simulink model "dspanc"  (Simulink 6.0)
settings: Solver=FixedStepDiscrete  StartTime=0.0  StopTime=7.87  RelTol=1e-3
StopFcn:
  | if exist('y_filtered','var'),
  |     soundsc(double(y_filtered),8000);
  | else uiwait(errordlg('You must run the simulation first.','Signal Processing Blockset Demo Error','modal'));
  | end
values from neighbouring files (symbols this model uses):
  D = var(Noisef)    [lmsxy.m]
undefined symbols (not defined in the file or in its folder): wavread
libraries: dspsnks4 x4, simulink x4, dspsrcs4 x2, dsparch4 x1, dspsigops x1, dspadpt3 x1
CloseFcn:
  | clear y_filtered y_noisy y_org;
settings Model: Creator=navan  LastModifiedBy=mkhan
settings DataIOCC: LimitDataPoints=off  SaveOutput=off  SaveTime=off  SignalLoggingName=sigsOut
settings OptimizationCC: InlineInvariantSignals=off
settings DebuggingCC: CheckExecutionContextPreStartOutputMsg=on  CheckExecutionContextRuntimeOutputMsg=on  SolverPrmCheckMsg=none  ParameterPrecisionLossMsg=none
settings HardwareCC: TargetUnknown=on
settings ModelReferenceCC: UpdateModelReferenceTargets=IfOutOfDate
settings SFSimCC: SFSimApplyToAllLibs=on  SFSimBuildMode=Incremental

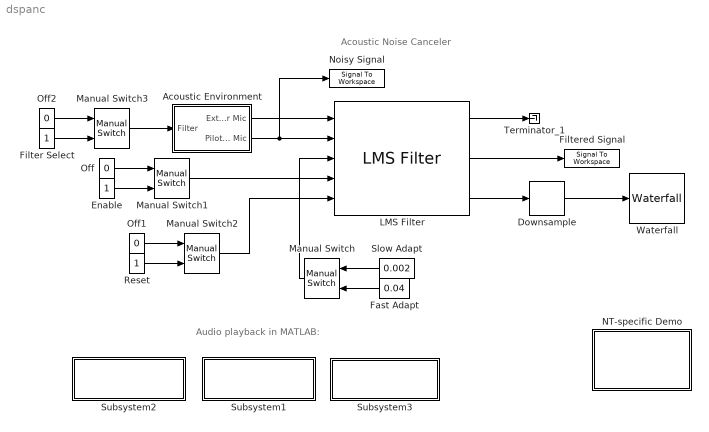
== system dspanc ==
  note: Acoustic Noise Canceler
  note: Audio playback in MATLAB:
  Acoustic Environment : Subsystem  PropExecContextAcrossSSBoundary=on
  Downsample : dspsigops/Downsample  N=32  phase=0  ic=0  smode=Allow multirate  fmode=Maintain input frame size
  Enable : Constant  OutDataTypeMode=boolean
  Fast Adapt : Constant  Orientation=left  Value=0.04
  Filter Select : Constant  OutDataTypeMode=boolean
  Filtered Signal : dspsnks4/Signal To Workspace  VariableName=y_filtered  FrameMode=Concatenate frames (2-D array)
      settings: FixptAsFi=off
  LMS Filter : dspadpt3/LMS Filter  DialogController=dspDDGCreate  DialogControllerArgs=DataTag1  Algo=Normalized LMS  L=40  stepflag=Input port  mu=0.1  leakage=1.0  ic=0  Adapt=on  resetflag=Non-zero sample  weights=on  secondCoeffMode=User-defined  secondCoeffWordLength=2  secondCoeffFracLength=15  accum2Mode=User-defined  accum2FracLength=20  prodOutput2Mode=User-defined  prodOutput2FracLength=20  prodOutput3Mode=User-defined  prodOutput3FracLength=20  prodOutput4Mode=User-defined  prodOutput4FracLength=20  quotientMode=User-defined  quotientFracLength=20  roundingMode=Floor  overflowMode=off  addnparflag=off
  Manual Switch : simulink/Signal Routing/Manual Switch  Orientation=left  sw=1  action=0
  Manual Switch1 : simulink/Signal Routing/Manual Switch  sw=0  action=0
  Manual Switch2 : simulink/Signal Routing/Manual Switch  sw=1  action=0
  Manual Switch3 : simulink/Signal Routing/Manual Switch  sw=1  action=0
  NT-specific Demo : Subsystem  PropExecContextAcrossSSBoundary=on
      settings: OpenFcn=dspanc_win32
      mask Type: NT-only Demo
      mask Display: disp('PC/Windows\nDemo')
  Noisy Signal : dspsnks4/Signal To Workspace  VariableName=y_noisy  FrameMode=Concatenate frames (2-D array)
      settings: FixptAsFi=off
  Off : Constant  Value=0  OutDataTypeMode=boolean
  Off1 : Constant  Value=0  OutDataTypeMode=boolean
  Off2 : Constant  Value=0  OutDataTypeMode=boolean
  Reset : Constant  OutDataTypeMode=boolean
  Slow Adapt : Constant  Orientation=left  Value=0.002
  Subsystem1 : Subsystem  PropExecContextAcrossSSBoundary=on
      settings: OpenFcn=if exist('y_noisy','var'), soundsc(double(y_noisy),8000); else uiwait(errordlg('You must run the simulation first.','Signal Processing Blockset Demo Error','modal')); end
      mask Display: disp('Noisy\nSignal')
  Subsystem2 : Subsystem  PropExecContextAcrossSSBoundary=on
      settings: OpenFcn=if exist('y_org','var'), soundsc(double(y_org)); else uiwait(errordlg('Data not found in workspace - run demo model.','Signal Processing Blockset Demo Error','modal'));end
      mask Display: disp('Original\nSignal')
  Subsystem3 : Subsystem  PropExecContextAcrossSSBoundary=on
      settings: OpenFcn=if exist('y_filtered','var'), soundsc(double(y_filtered),8000); else uiwait(errordlg('You must run the simulation first.','Signal Processing Blockset Demo Error','modal')); end
      mask Display: disp('Filtered\nSignal')
  Terminator_1 : Terminator
  Waterfall : dspsnks4/Waterfall  TraceProperties=off  NumTraces=6  CMapStr=autumn  TNewest=0.9  TOldest=0.5  HistoryLength=50  HistoryFull=Overwrite  UpdateInterval=1  ExportMode=All visible  MLExportName=ExportData  AutoExport=off  DisplayProperties=off  MouseMode=Orbit  AxisGrid=on  Snapshot=off  Suspend=off  SyncSnapshots=off  OpenScopeAtSimStart=off  FigPos=[27 57 405 339]  CameraView=[28.5695107359948 1316.8235109177 -294.350451091202 -0.004386576265097 22.5 3.5 0.594111941595966 -49.3321641526923 11.3523452384532 1.12783221137103 1 122.332173767783 16.310956502371]  InportDimsHint=[40 1]  AxisProperties=off  AxisColor='w'  XLabel=Amplitude  YLabel=Samples  ZLabel=Time  TriggerProperties=off  TrigStartMode=Immediately  TrigStartT=0  TrigStartN=0  TrigStartFcn=trigbegin  TrigStopMode=Never  TrigStopT=0.1  TrigStopN=1  TrigStopFcn=trigend  TrigRearmMode=Never  TrigRearmT=0  TrigRearmN=0  TrigRearmFcn=trigrearm  XformProperties=on  XformMode=None  XformFcn=abs  XformExpr=(u+1)/2
      settings: YMin=-0.188312025368214  YMax=0.17953887283802
  wires:
  Downsample/1 -> Waterfall/1
  Acoustic Environment/1(Exterior Mic) -> LMS Filter/1
  Slow Adapt/1 -> Manual Switch/1
  Fast Adapt/1 -> Manual Switch/2
  Manual Switch/1 -> LMS Filter/3
  LMS Filter/3 -> Downsample/1
  Acoustic Environment/2(Pilot's Mic) -> LMS Filter/2, Noisy Signal/1
  LMS Filter/2 -> Filtered Signal/1
  LMS Filter/1 -> Terminator_1/1
  Off/1 -> Manual Switch1/1
  Enable/1 -> Manual Switch1/2
  Off1/1 -> Manual Switch2/1
  Reset/1 -> Manual Switch2/2
  Manual Switch1/1 -> LMS Filter/4
  Manual Switch2/1 -> LMS Filter/5
  Off2/1 -> Manual Switch3/1
  Filter Select/1 -> Manual Switch3/2
  Manual Switch3/1 -> Acoustic Environment/1(Filter)

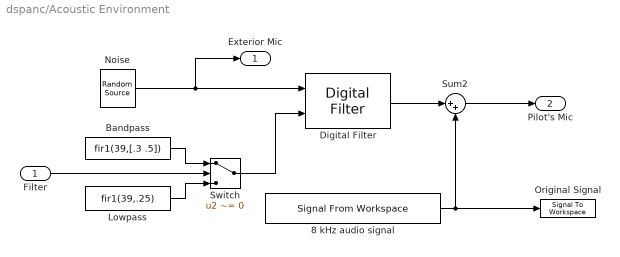
== system dspanc/Acoustic Environment ==
  Filter : Inport  LatchInput=off
  8 kHz audio signal : dspsrcs4/Signal From Workspace  X=single(wavread('dspafxf_8000.wav'))  Ts=1/8000  nsamps=32  OutputAfterFinalValue=Cyclic repetition
  Bandpass : Constant  Value=fir1(39,[.3 .5])
  Digital Filter : dsparch4/Digital Filter  DialogController=dspDDGCreate  DialogControllerArgs=DataTag0  TypePopup=FIR (all zeros)  IIRFiltStruct=Direct form II transposed  AllPoleFiltStruct=Direct form  FIRFiltStruct=Direct form  CoeffSource=Input port(s)  NumCoeffs=[1 2]  DenCoeffs=[1 0.1]  BiQuadCoeffs=[1 0.3 0.4 1 0.1 0.2]  LatticeCoeffs=[0.2 0.4]  denIgnore=on  FiltPerSampPopup=One filter per frame  IC=0  ICnum=0  ICden=0  roundingMode=Floor  overflowMode=off  ScaleValues=1  scaleValueFracLength=14  stageInFracLength=15  stageOutFracLength=15
  Lowpass : Constant  Value=fir1(39,.25)
  Noise : dspsrcs4/Random Source  SrcType=Gaussian  NormMethod=Sum of uniform values  CltLength=5  Min=-1  Max=1  Mean=0  Var=1  RepMode=Specify seed  rawSeed=[23341]  Inherit=off  SampMode=Discrete  SampTime=1/8000  SampFrame=32  DataType=Single  OutComplex=Real
  Original Signal : dspsnks4/Signal To Workspace  VariableName=y_org  FrameMode=Concatenate frames (2-D array)
      settings: FixptAsFi=off
  Sum2 : Sum  Inputs=|++  SaturateOnIntegerOverflow=on  InputSameDT=on
  Switch : Switch  Criteria=u2 ~= 0  SaturateOnIntegerOverflow=on
  Exterior Mic : Outport
  Pilot's Mic : Outport  Port=2
  wires:
  8 kHz audio signal/1 -> Sum2/2, Original Signal/1
  Sum2/1 -> Pilot's Mic/1
  Filter/1 -> Switch/2
  Digital Filter/1 -> Sum2/1
  Noise/1 -> Digital Filter/1, Exterior Mic/1
  Switch/1 -> Digital Filter/2
  Bandpass/1 -> Switch/1
  Lowpass/1 -> Switch/3

== system dspanc/NT-specific Demo ==

== system dspanc/Subsystem1 ==

== system dspanc/Subsystem2 ==

== system dspanc/Subsystem3 ==
